simulink model "Final_PAPER2_wtdelay_fuzzy"  (R2025b)
settings: Solver=ode23  StartTime=0.0  StopTime=8  RelTol=1e-3
undefined symbols (not defined in the file): A, B, sigbuilder_block
libraries: simulink_extras x4, fuzblock x1
settings Model: Creator=HP  LastModifiedBy=HP
settings OptimizationCC: ReuseModelBlockBuffer=off
settings RTWCC: GPUComputeCapability=3.5

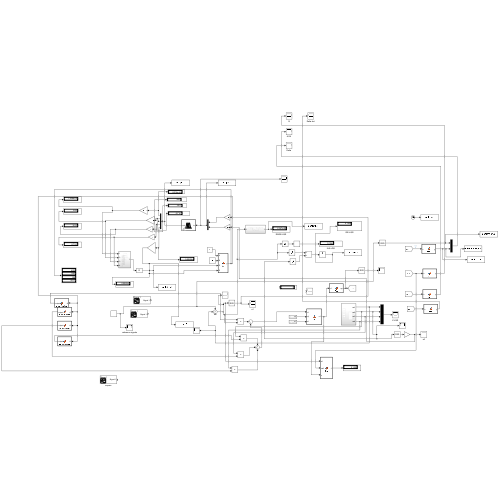
[thumbnail: Simulink's stored preview of the top-level diagram]
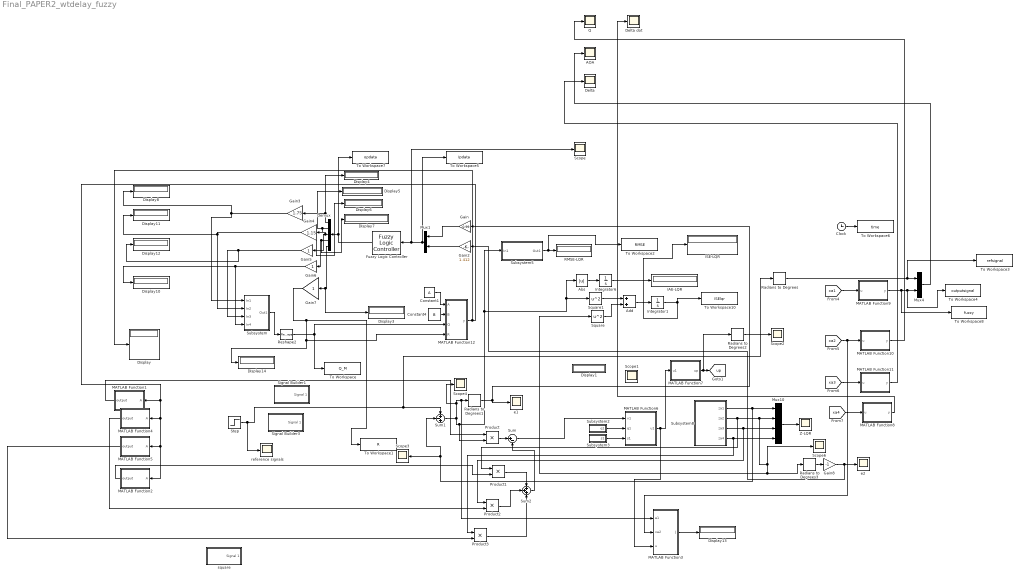
== system Final_PAPER2_wtdelay_fuzzy ==
  AOA : Scope
      settings: SampleTime=0.001  ActiveDisplayYMinimum=-1.91326  ActiveDisplayYMaximum=17.21938  DataLoggingVariableName=AOA_data
  Abs : Abs  SaturateOnIntegerOverflow=off
  Add : Sum
  Clock : Clock
  Constant1 : Constant  Value=A
  Constant4 : Constant  Value=B
  Delta : Scope
      settings: SampleTime=0.001  ActiveDisplayYMinimum=-21.856953764269463  ActiveDisplayYMaximum=2.4285504182521622  DataLoggingVariableName=Delta_data
  Delta dot : Scope
      settings: SampleTime=0.001  ActiveDisplayYMinimum=-52.861950793684656  ActiveDisplayYMaximum=7.85777152411853  DataLoggingVariableName=DeltaDot_data
  Demux : Demux  Outputs=5
  Display{,1,3..8,10..14} (13 alike) : Display
  Fuzzy Logic Controller : fuzblock/Fuzzy Logic  Controller  FIS='FLC_Final1.fis'  OutputSampleNumber=101  DataType=double  UseLookupTable=off  NumBreakpoints=10  FuzzifiedInputs=off  RuleFiringStrengths=off  RuleOutputs=off  AggregatedOutputs=off  SimulateUsing=Interpreted execution  OutOfRangeInputValueMessage=warning  NoRuleFiredMessage=warning  EmptyOutputFuzzySetMessage=warning
  Gain : Gain  Gain=0.99
  Gain2 : Gain  Gain=1.412
  Gain3 : Gain  Gain=1.75
  Gain4 : Gain  Gain=1.15
  Gain5 : Gain
  Gain6 : Gain
  Gain7 : Gain
  Gain8 : Gain  Gain=-1
  IAE-LQR : Display
  ISE-LQR : Display
  Integrator1 : Integrator
  Integrator6 : Integrator
  MATLAB Function1 : MATLAB Function  TreatAsAtomicUnit=on
  MATLAB Function10 : MATLAB Function  TreatAsAtomicUnit=on
  MATLAB Function11 : MATLAB Function  TreatAsAtomicUnit=on
  MATLAB Function12 : MATLAB Function  TreatAsAtomicUnit=on
  MATLAB Function2 : MATLAB Function  TreatAsAtomicUnit=on
  MATLAB Function3 : MATLAB Function  TreatAsAtomicUnit=on
  MATLAB Function4 : MATLAB Function  TreatAsAtomicUnit=on
  MATLAB Function5 : MATLAB Function  TreatAsAtomicUnit=on
  MATLAB Function6 : MATLAB Function  TreatAsAtomicUnit=on
  MATLAB Function7 : MATLAB Function  TreatAsAtomicUnit=on
  MATLAB Function8 : MATLAB Function  TreatAsAtomicUnit=on
  MATLAB Function9 : MATLAB Function  TreatAsAtomicUnit=on
  Mux1 : Mux  Inputs=2
  Mux10 : Mux
  Mux4 : Mux  Inputs=2
  Product{,1..3} (4 alike) : Product
  Q : Scope
      settings: SampleTime=0.001  ActiveDisplayYMinimum=-1  ActiveDisplayYMaximum=1  DataLoggingVariableName=Q_data
  RMSE-LQR : Display
  Radians to Degrees{,1..3} (4 alike) : simulink_extras/Transformations/Radians to Degrees
  Reshape2 : Reshape  OutputDimensionality=Customize  OutputDimensions=[4,4]
  Scope{,1..4,6} (6 alike) : Scope
      Scope settings: SampleTime=0.001  ActiveDisplayYMinimum=-1  ActiveDisplayYMaximum=1  DataLoggingVariableName=e1e2  DataLoggingSaveFormat=Array
      Scope1 settings: ActiveDisplayYMinimum=-9214.81546  ActiveDisplayYMaximum=17242.7377
      Scope2 settings: ActiveDisplayYMinimum=-21.84967  ActiveDisplayYMaximum=2.1717  DataLoggingVariableName=ScopeData3
      Scope3 settings: ActiveDisplayYMinimum=-0.34522  ActiveDisplayYMaximum=0.33356  DataLoggingVariableName=ScopeData2
      Scope4 settings: ActiveDisplayYMinimum=-0.29471  ActiveDisplayYMaximum=0.03442  DataLoggingVariableName=ScopeData3
      Scope6 settings: ActiveDisplayYMinimum=-3.06278  ActiveDisplayYMaximum=2.34785  DataLoggingVariableName=ScopeData4
  Signal Builder1 : Subsystem  Tag=STV Subsys  LoadFcn=sigbuilder_block('load');  StartFcn=sigbuilder_block('start');  StopFcn=sigbuilder_block('stop');  ClipboardFcn=sigbuilder_block('clipboard');  mask(Sigbuilder block){tuvar=[0:10]}
      mask help: Simulink:masks:SigbuilderBlock_MD
      mask init:
      | if ~strcmp(get_param(bdroot(gcbh),'SimulationStatus'),'stopped') tuvar = sigbuilder_block('maskInit'); end
      settings: CopyFcn=sigbuilder_block('copy');  DeleteFcn=sigbuilder_block('delete');  ModelCloseFcn=sigbuilder_block('modelClose');  PreSaveFcn=sigbuilder_block('preSave');  PauseFcn=sigbuilder_block('pause');  ContinueFcn=sigbuilder_block('continue');  NameChangeFcn=sigbuilder_block('namechange');  OpenFcn=sigbuilder_block('open',[5.4 -24.6 1141.2 477.6 ]);  CloseFcn=sigbuilder_block('close');
      mask Display: plot(0, 0, 100, 100,[2, 2, 32, 32, 2], [68, 8, 8, 68, 68],[32, 2], [38, 38], [32, 19, 2],[53, 60, 44], [32, 17, 17, 2],[16, 16, 31, 31]);txt = getActiveGroup(gcbh);text(2, 100, txt,'verticalAlignment', 'top');
  Signal Builder3 : Subsystem  Tag=STV Subsys  LoadFcn=sigbuilder_block('load');  StartFcn=sigbuilder_block('start');  StopFcn=sigbuilder_block('stop');  ClipboardFcn=sigbuilder_block('clipboard');  mask(Sigbuilder block){tuvar=[0:10]}
      mask help: Simulink:masks:SigbuilderBlock_MD
      mask init:
      | if ~strcmp(get_param(bdroot(gcbh),'SimulationStatus'),'stopped') tuvar = sigbuilder_block('maskInit'); end
      settings: CopyFcn=sigbuilder_block('copy');  DeleteFcn=sigbuilder_block('delete');  ModelCloseFcn=sigbuilder_block('modelClose');  PreSaveFcn=sigbuilder_block('preSave');  PauseFcn=sigbuilder_block('pause');  ContinueFcn=sigbuilder_block('continue');  NameChangeFcn=sigbuilder_block('namechange');  OpenFcn=sigbuilder_block('open',[5.4 -40.2 1141.2 515.4 ]);  CloseFcn=sigbuilder_block('close');
      mask Display: plot(0, 0, 100, 100,[2, 2, 32, 32, 2], [68, 8, 8, 68, 68],[32, 2], [38, 38], [32, 19, 2],[53, 60, 44], [32, 17, 17, 2],[16, 16, 31, 31]);txt = getActiveGroup(gcbh);text(2, 100, txt,'verticalAlignment', 'top');
  Square : Math  Operator=square
  Square1 : Math  Operator=square
  Step : Step  Time=0  After=0.2617795  SampleTime=0
  Subsystem : Subsystem
  Subsystem2 : Subsystem
  Subsystem3 : Subsystem
  Subsystem5 : Subsystem
  Subsystem8 : Subsystem
  Sum : Sum  Inputs=|+-
  Sum1 : Sum  Inputs=+-+
  Sum2 : Sum  Inputs=+++
  To Workspace : ToWorkspace  VariableName=Q_M  SampleTime=-1
  To Workspace1 : ToWorkspace  VariableName=R  SampleTime=-1
  To Workspace10 : ToWorkspace  VariableName=ISElqr  SampleTime=-1
  To Workspace2 : ToWorkspace  VariableName=RMSE  SampleTime=-1
  To Workspace3 : ToWorkspace  VariableName=refsignal  SampleTime=-1
  To Workspace4 : ToWorkspace  VariableName=outputsignal  SampleTime=-1
  To Workspace5 : ToWorkspace  VariableName=Ipdata  SampleTime=-1
  To Workspace6 : ToWorkspace  VariableName=time  SaveFormat=Timeseries  SampleTime=-1
  To Workspace7 : ToWorkspace  VariableName=opdata  SampleTime=-1
  To Workspace8 : ToWorkspace  VariableName=fuzzy  SaveFormat=Timeseries  SampleTime=-1
  Z-LQR : Scope
      settings: ActiveDisplayYMinimum=-319.11401  ActiveDisplayYMaximum=339.33228  DataLoggingVariableName=ScopeData2
  e1 : Scope
      settings: ActiveDisplayYMinimum=-37.64101  ActiveDisplayYMaximum=37.64545
  e2 : Scope
      settings: ActiveDisplayYMinimum=-133.21966  ActiveDisplayYMaximum=174.95549
  reference signals : Scope
      settings: ActiveDisplayYMinimum=-0.23071  ActiveDisplayYMaximum=0.31641
  square : Subsystem  Tag=STV Subsys  LoadFcn=sigbuilder_block('load');  StartFcn=sigbuilder_block('start');  StopFcn=sigbuilder_block('stop');  ClipboardFcn=sigbuilder_block('clipboard');  mask(Sigbuilder block){tuvar=[0:10]}
      mask help: Simulink:masks:SigbuilderBlock_MD
      mask init:
      | if ~strcmp(get_param(bdroot(gcbh),'SimulationStatus'),'stopped') tuvar = sigbuilder_block('maskInit'); end
      settings: CopyFcn=sigbuilder_block('copy');  DeleteFcn=sigbuilder_block('delete');  ModelCloseFcn=sigbuilder_block('modelClose');  PreSaveFcn=sigbuilder_block('preSave');  PauseFcn=sigbuilder_block('pause');  ContinueFcn=sigbuilder_block('continue');  NameChangeFcn=sigbuilder_block('namechange');  OpenFcn=sigbuilder_block('open',[5.4 36 1141.2 516.6 ]);  CloseFcn=sigbuilder_block('close');
      mask Display: plot(0, 0, 100, 100,[2, 2, 32, 32, 2], [68, 8, 8, 68, 68],[32, 2], [38, 38], [32, 19, 2],[53, 60, 44], [32, 17, 17, 2],[16, 16, 31, 31]);txt = getActiveGroup(gcbh);text(2, 100, txt,'verticalAlignment', 'top');
  tag scope: up=global
  wires:
  [xa4] -> MATLAB Function8/1(u)
  Subsystem2/1(q1) -> MATLAB Function6/2(q1)
  Subsystem3/1(s1) -> MATLAB Function6/3(s1)
  MATLAB Function6/1(u1) -> MATLAB Function3/3(u), MATLAB Function7/1(u1)
  [xa3] -> MATLAB Function11/1(u)
  [xa2] -> MATLAB Function3/2(xa2), MATLAB Function10/1(u)
  MATLAB Function10/1(y) -> Q/1
  MATLAB Function11/1(y) -> Delta/1
  [xa1] -> MATLAB Function9/1(u)
  Mux4/1 -> AOA/1
  Integrator1/1 -> To Workspace10/1, ISE-LQR/1
  Subsystem5/1(Out1) -> To Workspace2/1, RMSE-LQR/1
  Sum1/1 -> Scope4/1, MATLAB Function3/1(e1), Radians to Degrees1/1, Product/2, Square1/1, Abs/1, Subsystem5/1(In1)
  Abs/1 -> Integrator6/1
  Integrator6/1 -> IAE-LQR/1
  MATLAB Function7/1(up) -> Radians to Degrees2/1, [up]
  Mux10/1 -> Z-LQR/1
  Subsystem8/4(za4) -> Product3/1, Mux10/4
  Subsystem8/3(za3) -> Product2/1, Mux10/3
  Subsystem8/1(za1) -> Sum1/2, Scope3/1, Mux10/1
  MATLAB Function9/1(y) -> To Workspace8/1, To Workspace4/1, Mux4/2
  MATLAB Function8/1(y) -> Delta dot/1
  Radians to Degrees/1 -> To Workspace3/1, Mux4/1
  Clock/1 -> To Workspace6/1
  Gain/1 -> Mux1/1
  Gain2/1 -> Mux1/2
  Mux1/1 -> To Workspace5/1, Scope/1, Fuzzy Logic Controller/1
  Fuzzy Logic Controller/1 -> Demux/1, To Workspace7/1
  Gain3/1 -> Subsystem/1(In1), Display8/1
  Gain4/1 -> Display11/1, Subsystem/2(In2)
  Gain5/1 -> Display12/1, Subsystem/3(In3)
  Subsystem/1(Out1) -> Reshape2/1
  Radians to Degrees1/1 -> Gain/1, e1/1
  Radians to Degrees2/1 -> Scope2/1
  Subsystem8/2(za2) -> Product1/1, Scope6/1, Radians to Degrees3/1, Square/1, Mux10/2
  Radians to Degrees3/1 -> Gain8/1
  Gain8/1 -> Gain2/1, e2/1
  Gain6/1 -> Display10/1, Subsystem/4(In4)
  Add/1 -> Integrator1/1
  Square/1 -> Add/2
  Square1/1 -> Add/1
  MATLAB Function3/1(J) -> Display13/1
  Sum2/1 -> Sum/2
  Sum/1 -> MATLAB Function6/1(v1)
  Step/1 -> reference signals/1, Radians to Degrees/1, Sum1/1
  Gain7/1 -> Display14/1, MATLAB Function12/4(R), To Workspace1/1
  Reshape2/1 -> To Workspace/1, MATLAB Function12/3(Q)
  MATLAB Function12/1(y) -> MATLAB Function2/1(A), MATLAB Function5/1(A), MATLAB Function4/1(A), MATLAB Function1/1(A), Display/1
  Constant4/1 -> MATLAB Function12/2(B)
  Constant1/1 -> MATLAB Function12/1(A)
  MATLAB Function1/1(output) -> Product/1
  Product/1 -> Sum/1
  MATLAB Function2/1(output) -> Product1/2
  Product1/1 -> Sum2/1
  MATLAB Function4/1(output) -> Product2/2
  Product2/1 -> Sum2/2
  MATLAB Function5/1(output) -> Product3/2
  Product3/1 -> Sum2/3
  Demux/1 -> Display4/1, Gain3/1
  Demux/2 -> Display5/1, Gain4/1
  Demux/3 -> Display6/1, Gain5/1
  Demux/4 -> Display7/1, Gain6/1
  Demux/5 -> Display3/1, Gain7/1

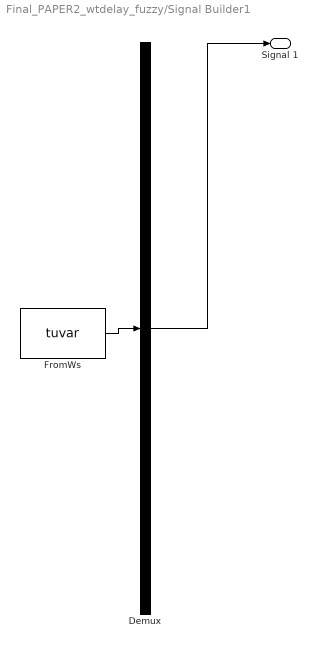
== system Final_PAPER2_wtdelay_fuzzy/Signal Builder1 ==
  Demux : Demux  Tag=STV Demux  Outputs=1
      settings: DisplayOption=none
  FromWs : FromWorkspace  Tag=STV FromWs  VariableName=tuvar
      SigBuilderData=|
      | common.afterFinalStr = 'Extrapolate'
      | common.sampleTime = 0
      | dataSet.timeRange = [0 10]
      | dataSet.name = 'Group 1'
      | sbobj.Groups.Name = 'Group 1'
      | sbobj.Groups.Signals.Name = 'Signal 1'
      | sbobj.Groups.Signals.XData = [0 2 2 4 4 6 6 8 8 10]
      | sbobj.Groups.Signals.YData = [-0.176 -0.176 0.176 0.176 -0.176 -0.176 0.176 0.176 -0.176 -0.176]
  Signal 1 : Outport  Tag=STV Outport
  wires:
  Demux/1 -> Signal 1/1
  FromWs/1 -> Demux/1

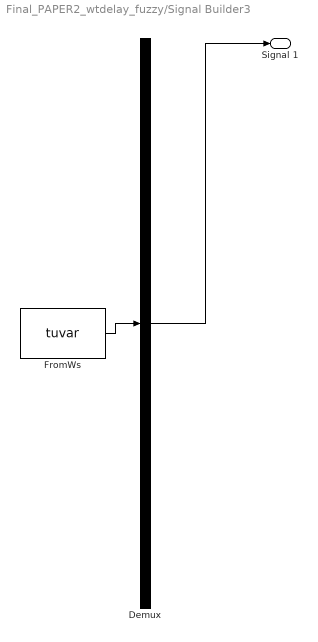
== system Final_PAPER2_wtdelay_fuzzy/Signal Builder3 ==
  Demux : Demux  Tag=STV Demux  Outputs=1
      settings: DisplayOption=none
  FromWs : FromWorkspace  Tag=STV FromWs  VariableName=tuvar
      SigBuilderData=|
      | common.afterFinalStr = 'Extrapolate'
      | common.sampleTime = 0
      | dataSet.timeRange = [0 6]
      | dataSet.name = 'Group 1'
      | sbobj.Groups.Name = 'Group 1'
      | sbobj.Groups.Signals.Name = 'Signal 1'
      | sbobj.Groups.Signals.XData = [0 2 2 4 4 6]
      | sbobj.Groups.Signals.YData = [0.261799 0.261799 -0.261799 -0.261799 0.261799 0.261799]
      | sbobj.Groups.TimeRange = [0 6]
  Signal 1 : Outport  Tag=STV Outport
  wires:
  Demux/1 -> Signal 1/1
  FromWs/1 -> Demux/1

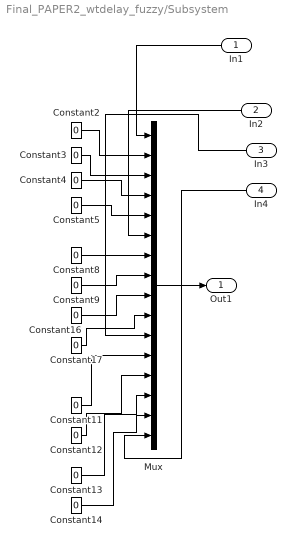
== system Final_PAPER2_wtdelay_fuzzy/Subsystem ==
  In1 : Inport
  In2 : Inport  Port=2
  In3 : Inport  Port=3
  In4 : Inport  Port=4
  Constant{2..5,8..9,11..14,16..17} (12 alike) : Constant  Value=0
  Mux : Mux  Inputs=16
  Out1 : Outport
  wires:
  Constant8/1 -> Mux/7
  Constant4/1 -> Mux/4
  Constant2/1 -> Mux/2
  In4/1 -> Mux/16
  Constant5/1 -> Mux/5
  Constant17/1 -> Mux/10
  Constant12/1 -> Mux/13
  Constant9/1 -> Mux/8
  Constant13/1 -> Mux/14
  Constant11/1 -> Mux/12
  Constant14/1 -> Mux/15
  Constant3/1 -> Mux/3
  Constant16/1 -> Mux/9
  In2/1 -> Mux/6
  In3/1 -> Mux/11
  In1/1 -> Mux/1
  Mux/1 -> Out1/1

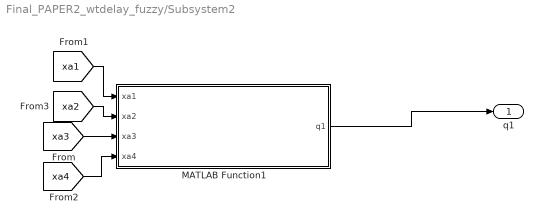
== system Final_PAPER2_wtdelay_fuzzy/Subsystem2 ==
  MATLAB Function1 : MATLAB Function  TreatAsAtomicUnit=on
  q1 : Outport
  wires:
  [xa2] -> MATLAB Function1/2(xa2)
  [xa1] -> MATLAB Function1/1(xa1)
  MATLAB Function1/1(q1) -> q1/1
  [xa3] -> MATLAB Function1/3(xa3)
  [xa4] -> MATLAB Function1/4(xa4)

== system Final_PAPER2_wtdelay_fuzzy/Subsystem3 ==
  MATLAB Function5 : MATLAB Function  TreatAsAtomicUnit=on
  Scope : Scope
      settings: ActiveDisplayYMinimum=-11135.15313  ActiveDisplayYMaximum=-11030.38049  DataLoggingVariableName=ScopeData2
  s1 : Outport
  wires:
  MATLAB Function5/1(s1) -> Scope/1, s1/1

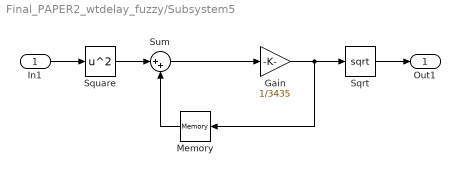
== system Final_PAPER2_wtdelay_fuzzy/Subsystem5 ==
  In1 : Inport
  Gain : Gain  Gain=1/3435
  Memory : Memory
  Sqrt : Sqrt
  Square : Math  Operator=square
  Sum : Sum  Inputs=|++
  Out1 : Outport
  wires:
  In1/1 -> Square/1
  Square/1 -> Sum/1
  Memory/1 -> Sum/2
  Sum/1 -> Gain/1
  Gain/1 -> Sqrt/1, Memory/1
  Sqrt/1 -> Out1/1

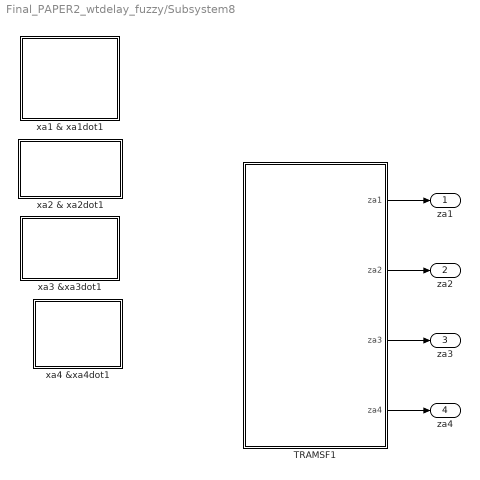
== system Final_PAPER2_wtdelay_fuzzy/Subsystem8 ==
  " xa3 &xa3dot1" : Subsystem
  TRAMSF1 : Subsystem
  xa1 & xa1dot1 : Subsystem
  xa2 & xa2dot1 : Subsystem
  xa4 &xa4dot1 : Subsystem
  za1 : Outport
  za2 : Outport  Port=2
  za3 : Outport  Port=3
  za4 : Outport  Port=4
  wires:
  TRAMSF1/1(za1) -> za1/1
  TRAMSF1/3(za3) -> za3/1
  TRAMSF1/2(za2) -> za2/1
  TRAMSF1/4(za4) -> za4/1

== system Final_PAPER2_wtdelay_fuzzy/square ==
  Demux : Demux  Tag=STV Demux  Outputs=1
      settings: DisplayOption=none
  FromWs : FromWorkspace  Tag=STV FromWs  VariableName=tuvar
      SigBuilderData=|
      | common.afterFinalStr = 'Extrapolate'
      | common.sampleTime = 0
      | dataSet.timeRange = [0 10]
      | dataSet.name = 'Group 1'
      | sbobj.Groups.Name = 'Group 1'
      | sbobj.Groups.Signals.Name = 'Signal 1'
      | sbobj.Groups.Signals.XData = [0 2 2 4 4 10]
      | sbobj.Groups.Signals.YData = [0.2617 0.2617 -0.176 -0.176 0.176 0.176]
  Signal 1 : Outport  Tag=STV Outport
  wires:
  Demux/1 -> Signal 1/1
  FromWs/1 -> Demux/1

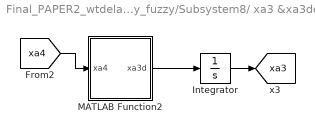
== system Final_PAPER2_wtdelay_fuzzy/Subsystem8/ xa3 &xa3dot1 ==
  Integrator : Integrator
  MATLAB Function2 : MATLAB Function  TreatAsAtomicUnit=on
  tag scope: xa3=global
  wires:
  Integrator/1 -> [xa3]
  [xa4] -> MATLAB Function2/1(xa4)
  MATLAB Function2/1(xa3d) -> Integrator/1

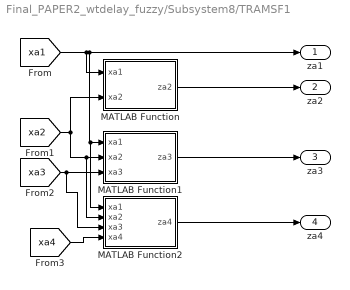
== system Final_PAPER2_wtdelay_fuzzy/Subsystem8/TRAMSF1 ==
  MATLAB Function : MATLAB Function  TreatAsAtomicUnit=on
  MATLAB Function1 : MATLAB Function  TreatAsAtomicUnit=on
  MATLAB Function2 : MATLAB Function  TreatAsAtomicUnit=on
  za1 : Outport
  za2 : Outport  Port=2
  za3 : Outport  Port=3
  za4 : Outport  Port=4
  wires:
  [xa1] -> MATLAB Function2/1(xa1), MATLAB Function1/1(xa1), za1/1, MATLAB Function/1(xa1)
  [xa2] -> MATLAB Function2/2(xa2), MATLAB Function1/2(xa2), MATLAB Function/2(xa2)
  MATLAB Function/1(za2) -> za2/1
  [xa3] -> MATLAB Function2/3(xa3), MATLAB Function1/3(xa3)
  MATLAB Function1/1(za3) -> za3/1
  [xa4] -> MATLAB Function2/4(xa4)
  MATLAB Function2/1(za4) -> za4/1

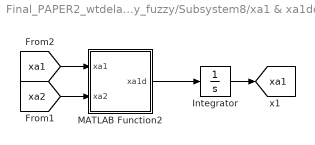
== system Final_PAPER2_wtdelay_fuzzy/Subsystem8/xa1 & xa1dot1 ==
  Integrator : Integrator
  MATLAB Function2 : MATLAB Function  TreatAsAtomicUnit=on
  tag scope: xa1=global
  wires:
  Integrator/1 -> [xa1]
  [xa1] -> MATLAB Function2/1(xa1)
  MATLAB Function2/1(xa1d) -> Integrator/1
  [xa2] -> MATLAB Function2/2(xa2)

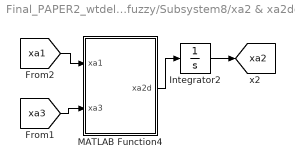
== system Final_PAPER2_wtdelay_fuzzy/Subsystem8/xa2 & xa2dot1 ==
  Integrator2 : Integrator
  MATLAB Function4 : MATLAB Function  TreatAsAtomicUnit=on
  tag scope: xa2=global
  wires:
  MATLAB Function4/1(xa2d) -> Integrator2/1
  Integrator2/1 -> [xa2]
  [xa3] -> MATLAB Function4/2(xa3)
  [xa1] -> MATLAB Function4/1(xa1)

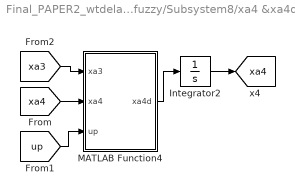
== system Final_PAPER2_wtdelay_fuzzy/Subsystem8/xa4 &xa4dot1 ==
  Integrator2 : Integrator
  MATLAB Function4 : MATLAB Function  TreatAsAtomicUnit=on
  tag scope: xa4=global
  wires:
  MATLAB Function4/1(xa4d) -> Integrator2/1
  Integrator2/1 -> [xa4]
  [xa3] -> MATLAB Function4/1(xa3)
  [up] -> MATLAB Function4/3(up)
  [xa4] -> MATLAB Function4/2(xa4)

== matlab function Final_PAPER2_wtdelay_fuzzy/MATLAB Function9 ==
  data: u input; y output
function y = fcn(u)

y = u*57.32;

== matlab function Final_PAPER2_wtdelay_fuzzy/Subsystem2/MATLAB Function1 ==
  data: q1 output; xa1 input; xa2 input; xa3 input; xa4 input
function q1 = fcn(xa1,xa2,xa3,xa4)
an=0.000103;
bn=-0.00945;
cn=-0.1696;
dn=-0.034;
am=0.000215;
bm=-0.0195;
cm=0.051;
dm=-0.206;
k=57.3248;
Kq=1.23202439;
Ka=0.020691432;
M=2.5;
wa=50;
zt = 1.4;
q1=dm*k*Kq*M^2*(-wa^2*xa3-wa*xa4*zt) + dm*k*Kq*M^2*xa4*(Ka*M*cos(xa1)*(cn*k*(2-M/3)+ 3*an*k^3*xa1^2+2*bn*k^2*abs(xa1))-Ka*M*(cn*k*(2-M/3)*xa1+an*k^3*xa1^3+bn*k^2*xa1*abs(xa1))*sin(xa1))+Kq*M^2*(cm*k*(-7 + (8*M)/3)*xa1 + am*k^3*xa1^3 + dm*k*xa3 + bm*k^2*xa1*abs(xa1))*(Kq*M^2*(cm*k*(-7 + (8*M)/3) +3*am*k^3*xa1^2 +2* bm*k^2*abs(xa1)) + 2*(xa2 + Ka*M*cos(xa1)*(cn*k*(2-M/3)*xa1 + an*k^3*xa1^3 +bn*k^2*xa1*abs(xa1)))*(Ka*M*cos(xa1)*(6*an*k^3*xa1 - bn*k^2*sign(xa1) + 3*bn*k^2*sign(xa1)) - Ka*M*cos(xa1)*(cn*k*(2-M/3)*xa1 + an*k^3*xa1^3 + bn*k^2*xa1*abs(xa1)) - 2*Ka*M*(cn*k*(2-M/3) + 3*an*k^3*xa1^2 + 2*bn*k^2*abs(xa1))*sin(xa1)) + (Ka*M*cos(xa1)*(cn*k*(2-M/3) + 3*an*k^3*xa1^2 + 2*bn*k^2*abs(xa1)) - Ka*M*(cn*k*(2-M/3)*xa1 + an*k^3*xa1^3 + bn*k^2*xa1*abs(xa1))*sin(xa1))^2) + (xa2 + Ka*M*cos(xa1)*(cn*k*(2-M/3)*xa1 + an*k^3*xa1^3 + bn*k^2*xa1*abs(xa1)))*(Kq*M^2*(cm*k*(-7 + (8*M)/3)*xa1 + am*k^3*xa1^3 + dm*k*xa3 + bm*k^2*xa1*abs(xa1))*(Ka*M*cos(xa1)*(6*an*k^3*xa1 - bn*k^2*sign(xa1) + 3*bn*k^2*sign(xa1))-Ka*M*cos(xa1)*(cn*k*(2-M/3)*xa1+an*k^3*xa1^3+bn*k^2*xa1*abs(xa1))-2*Ka*M*(cn*k*(2-M/3)+3*an*k^3*xa1^2+2*bn*k^2*abs(xa1))*sin(xa1))+ Kq*M^2*(cm*k*(-7+(8*M)/3)+3*am*k^3*xa1^2+2*bm*k^2*abs(xa1))*(Ka*M*cos(xa1)*(cn*k*(2-M/3)+3*an*k^3*xa1^2+2*bn*k^2*abs(xa1)) - Ka*M*(cn*k*(2-M/3)*xa1+an*k^3*xa1^3+bn*k^2*xa1*abs(xa1))*sin(xa1))+(Ka*M*cos(xa1)*(cn*k*(2-M/3)+3*an*k^3*xa1^2+2*bn*k^2*abs(xa1)) - Ka*M*(cn*k*(2-M/3)*xa1+an*k^3*xa1^3+bn*k^2*xa1*abs(xa1))*sin(xa1))*(Kq*M^2*(cm*k*(-7+(8*M)/3)+3*am*k^3*xa1^2+2*bm*k^2*abs(xa1))+(xa2 + Ka*M*cos(xa1)*(cn*k*(2-M/3)*xa1+an*k^3*xa1^3+bn*k^2*xa1*abs(xa1)))*(Ka*M*cos(xa1)*(6*an*k^3*xa1 - bn*k^2*sign(xa1) + 3*bn*k^2*sign(xa1))-Ka*M*cos(xa1)*(cn*k*(2-M/3)*xa1+an*k^3*xa1^3+bn*k^2*xa1*abs(xa1))-2*Ka*M*(cn*k*(2-M/3) + 3*an*k^3*xa1^2 + 2*bn*k^2*abs(xa1))*sin(xa1))+(Ka*M*cos(xa1)*(cn*k*(2-M/3) + 3*an*k^3*xa1^2 + 2*bn*k^2*abs(xa1)) - Ka*M*(cn*k*(2-M/3)*xa1 + an*k^3*xa1^3 + bn*k^2*xa1*abs(xa1))*sin(xa1))^2)+(xa2 + Ka*M*cos(xa1)*(cn*k*(2-M/3)*xa1 + an*k^3*xa1^3 +bn*k^2*xa1*abs(xa1)))*(Kq*M^2*(6*am*k^3*xa1-bm*k^2*sign(xa1)+3*bm*k^2*sign(xa1)) + 3*(Ka*M*cos(xa1)*(6*an*k^3*xa1-bn*k^2*sign(xa1)+3*bn*k^2*sign(xa1)) - Ka*M*cos(xa1)*(cn*k*(2-M/3)*xa1+an*k^3*xa1^3+bn*k^2*xa1*abs(xa1)) - 2*Ka*M*(cn*k*(2-M/3)+3*an*k^3*xa1^2+2*bn*k^2*abs(xa1))*sin(xa1))*(Ka*M*cos(xa1)*(cn*k*(2-M/3)+3*an*k^3*xa1^2+2*bn*k^2*abs(xa1)) - Ka*M*(cn*k*(2-M/3)*xa1+an*k^3*xa1^3+bn*k^2*xa1*abs(xa1))*sin(xa1))+(xa2 + Ka*M*cos(xa1)*(cn*k*(2-M/3)*xa1+an*k^3*xa1^3+bn*k^2*xa1*abs(xa1)))*(Ka*M*cos(xa1)*6*an*k^3-3*Ka*M*cos(xa1)*(cn*k*(2-M/3)+3*an*k^3*xa1^2+2*bn*k^2*abs(xa1))-3*Ka*M*(6*an*k^3*xa1-bn*k^2*sign(xa1)+3*bn*k^2*sign(xa1))*sin(xa1)+Ka*M*(cn*k*(2-M/3)*xa1+an*k^3*xa1^3+bn*k^2*xa1*abs(xa1))*sin(xa1))));

== matlab function Final_PAPER2_wtdelay_fuzzy/Subsystem3/MATLAB Function5 ==
  data: s1 output
function s1 = fcn()
an=0.000103;
bn=-0.00945;
cn=-0.1696;
dn=-0.034;
am=0.000215;
bm=-0.0195;
cm=0.051;
dm=-0.206;
k=57.32;
wa=50;
Kq=1.23202439;
em=-0.03000221;
M=2.5;
s1=Kq*dm*k*wa^2*M^2;

== matlab function Final_PAPER2_wtdelay_fuzzy/Subsystem8/TRAMSF1/MATLAB Function ==
  data: xa1 input; za2 output; xa2 input
function za2 = fcn(xa1,xa2)
an=0.000103;
bn=-0.00945;
cn=-0.1696;
dn=-0.034;
am=0.000215;
bm=-0.0195;
cm=0.051;
dm=-0.206;
k=57.3248;
em=-0.03000221;
Kq=1.23202439;
Ka=0.020691432;
M=2.5;
wa=50;
za2 = xa2 + k*Ka*M*xa1*cos(xa1) * (-1/3*cn*(-6+M) + an*k^2*xa1^2 + bn*k*abs(xa1));

== matlab function Final_PAPER2_wtdelay_fuzzy/Subsystem8/TRAMSF1/MATLAB Function1 ==
  data: xa1 input; za3 output; xa2 input; xa3 input
function za3 = fcn(xa1,xa2,xa3)
an=0.000103;
bn=-0.00945;
cn=-0.1696;
dn=-0.034;
am=0.000215;
bm=-0.0195;
cm=0.051;
dm=-0.206;
k=57.3248;
em=-0.03000221;
Kq=1.23202439;
Ka=0.020691432;
M=2.5;
wa=50;
za3=M*(k*Kq*M*(cm*(-7 + (8*M)/3)*xa1 + am*k^2*xa1^3 + dm*xa3 + bm*k*xa1*abs(xa1)) + Ka*(xa2 + k*Ka*M*xa1*cos(xa1)*(-(1/3)*cn*(-6 + M) + an*k^2*xa1^2 + bn*k*abs(xa1)))*(k*cos(xa1)*(-(1/3)*cn*(-6 + M) + 3*an*k^2*xa1^2 + 2*bn*k*abs(xa1)) + (1/3)*k*xa1*(cn*(-6 + M) - 3*an*k^2*xa1^2 - 3*bn*k*abs(xa1))*sin(xa1)));

== matlab function Final_PAPER2_wtdelay_fuzzy/Subsystem8/TRAMSF1/MATLAB Function2 ==
  data: xa1 input; za4 output; xa2 input; xa3 input; xa4 input
function za4 = fcn(xa1,xa2,xa3,xa4)
an=0.000103;
bn=-0.00945;
cn=-0.1696;
dn=-0.034;
am=0.000215;
bm=-0.0195;
cm=0.051;
dm=-0.206;
k=57.3248;
em=-0.03000221;
Kq=1.23202439;
Ka=0.020691432;
M=2.5;
wa=50;
za4 = dm*k*Kq*M^2*xa4 + Kq*M^2*(cm*k*(-7 + (8*M)/3)*xa1 + am*k^3*xa1^3 + dm*k*xa3 + bm*k^2*xa1*abs(xa1))*(Ka*M*cos(xa1)*(cn*k*(2 - M/3) + 3*an*k^3*xa1^2 + bn*k^2*abs(xa1) + bn*k^2*abs(xa1))-Ka*M*(cn*k*(2 - M/3)*xa1 + an*k^3*xa1^3 + bn*k^2*xa1*abs(xa1))*sin(xa1)) + (xa2 + Ka*M*cos(xa1)*(cn*k*(2 - M/3)*xa1 + an*k^3*xa1^3 + bn*k^2*xa1*abs(xa1)))*(Kq*M^2*(cm*k*(-7 + (8*M)/3) + 3*am*k^3*xa1^2 + bm*k^2*abs(xa1) + bm*k^2*abs(xa1))+(xa2 + Ka*M*cos(xa1)*(cn*k*(2 - M/3)*xa1 + an*k^3*xa1^3 + bn*k^2*xa1*abs(xa1)))*(Ka*M*cos(xa1)*(6*an*k^3*xa1 - (bn*k^2*sign(xa1)) + 3*bn*k^2*sign(xa1))-Ka*M*cos(xa1)*(cn*k*(2 - M/3)*xa1 + an*k^3*xa1^3 + bn*k^2*xa1*abs(xa1))-2*Ka*M*(cn*k*(2 - M/3) + 3*an*k^3*xa1^2 + bn*k^2*abs(xa1) + bn*k^2*abs(xa1))*sin(xa1))+(Ka*M*cos(xa1)*(cn*k*(2 - M/3) + 3*an*k^3*xa1^2 + bn*k^2*abs(xa1) + bn*k^2*abs(xa1))-Ka*M*(cn*k*(2 - M/3)*xa1 + an*k^3*xa1^3 + bn*k^2*xa1*abs(xa1))*sin(xa1))^2);

== matlab function Final_PAPER2_wtdelay_fuzzy/MATLAB Function1 ==
  data: A input; output output
function output = extractValue(A)
    output = A(1, 1); 
end

== matlab function Final_PAPER2_wtdelay_fuzzy/Subsystem8/xa1 & xa1dot1/MATLAB Function2 ==
  data: xa1 input; xa1d output; xa2 input
function xa1d = fcn(xa1,xa2)
an=0.000103;
bn=-0.00945;
cn=-0.1696;
dn=-0.034;
am=0.000215;
bm=-0.0195;
cm=0.051;
dm=-0.206;
k=180/pi;
Ka=0.020691432;
Kq=1.23202439;
em=-0.03000221;
M=2.5;
wa=50;
xa1d=Ka*M*(an*xa1^3*k^3 + bn*xa1*abs(xa1)*k^2 + cn*(2 - (M/3))*xa1*k)*cos(xa1) + xa2;

== matlab function Final_PAPER2_wtdelay_fuzzy/Subsystem8/xa2 & xa2dot1/MATLAB Function4 ==
  data: xa1 input; xa2d output; xa3 input
function xa2d = fcn(xa1,xa3)
an=0.000103;
bn=-0.00945;
cn=-0.1696;
dn=-0.034;
am=0.000215;
bm=-0.0195;
cm=0.051;
dm=-0.206;
k=57.3248;
Ka=0.020691432;
Kq=1.23202439;
em=-0.03000221;
M=2.5;
wa=50;
xa2d=Kq*M^2*(am*xa1^3*k^3 + bm*xa1*abs(xa1)*k^2 + cm*(-7 + (8*M/3))*xa1*k + dm*k*xa3);

== matlab function Final_PAPER2_wtdelay_fuzzy/Subsystem8/xa4 &xa4dot1/MATLAB Function4 ==
  data: xa3 input; xa4 input; xa4d output; up input
function xa4d = fcn(xa3,xa4,up)
an=0.000103;
bn=-0.00945;
cn=-0.1696;
dn=-0.034;
am=0.000215;
bm=-0.0195;
cm=0.051;
dm=-0.206;
k=57.3248;
em=-0.03000221;
M=2.5;
wa=50;
zt=1.4
xa4d= -wa^2*xa3 -zt*wa*xa4 + wa^2*up;

== matlab function Final_PAPER2_wtdelay_fuzzy/MATLAB Function3 ==
  data: e1 input; J output; xa2 input; u input
function  J = fcn(e1,xa2,u)

J=e1*e1+xa2*xa2+u*u;

== matlab function Final_PAPER2_wtdelay_fuzzy/MATLAB Function12 ==
  data: A input; y output; B input; Q input; R input
function y = fcn(A,B,Q,R)
y = zeros(1,4);
coder.extrinsic('lqr');
y = lqr(A,B,Q,R);

== matlab function Final_PAPER2_wtdelay_fuzzy/Subsystem8/ xa3 &xa3dot1/MATLAB Function2 ==
  data: xa4 input; xa3d output
function xa3d = fcn(xa4)
xa3d=xa4;

== matlab function Final_PAPER2_wtdelay_fuzzy/MATLAB Function2 ==
  data: A input; output output
function output = extractValue(A)
    output = A(1, 2); 
end

== matlab function Final_PAPER2_wtdelay_fuzzy/MATLAB Function10 ==
  data: u input; y output
function y = fcn(u)

y = u*57.32;

== matlab function Final_PAPER2_wtdelay_fuzzy/MATLAB Function4 ==
  data: A input; output output
function output = extractValue(A)
    output = A(1, 3); 
end

== matlab function Final_PAPER2_wtdelay_fuzzy/MATLAB Function5 ==
  data: A input; output output
function output = extractValue(A)
    output = A(1,4 ...
        ); 
end

== matlab function Final_PAPER2_wtdelay_fuzzy/MATLAB Function11 ==
  data: u input; y output
function y = fcn(u)

y = u*57.32;

== matlab function Final_PAPER2_wtdelay_fuzzy/MATLAB Function6 ==
  data: v1 input; u1 output; q1 input; s1 input
function u1 = fcn(v1,q1,s1)
u1 = (v1-q1)/s1;

== matlab function Final_PAPER2_wtdelay_fuzzy/MATLAB Function7 ==
  data: u1 input; up output
function up = fcn(u1)

up = u1;

== matlab function Final_PAPER2_wtdelay_fuzzy/MATLAB Function8 ==
  data: u input; y output
function y = fcn(u)

y = u*57.32;
